simulink library "MarIn_blade"  (R2017a)
settings: Solver=VariableStepAuto  StartTime=0.0  StopTime=10.0  RelTol=1e-3
undefined symbols (not defined in the file or in its folder): bladePar, data_wind_mann, eta_init_n, g, k_t1, k_t2, k_w1, k_w2, lw2, m_h, meanWindSpeed, nu_init_b, p_h_dot_init, p_h_init, posCraneTip, posSling_b, posTuggerline_b, posTuggerlineBase_n, sigbuilder_block
undefined symbols (not defined in the file): d_w1, lt1_init
libraries: MarIn_blade x37
(part 2 of 2)

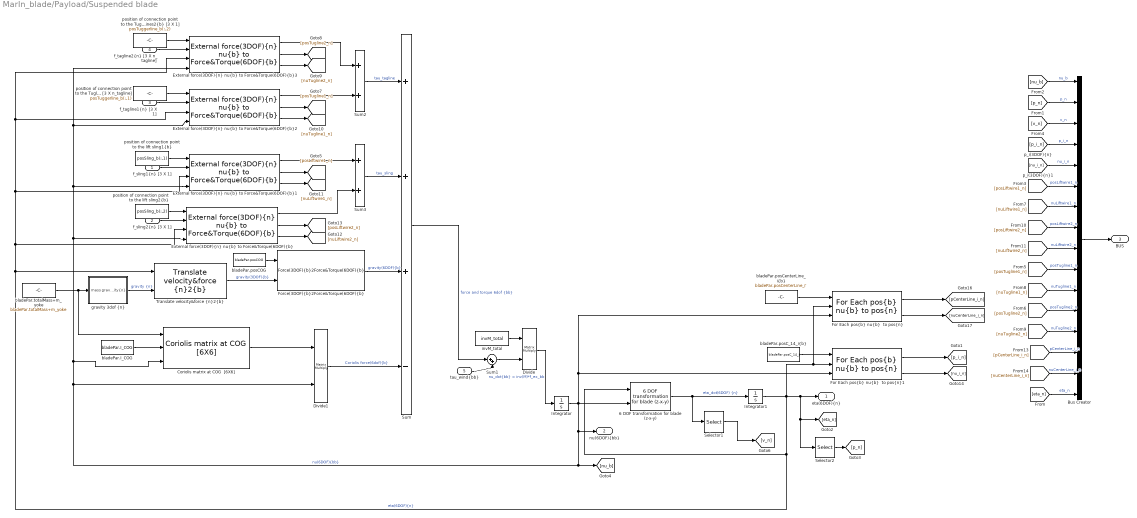
== system MarIn_blade/Payload/Suspended blade ==
  "f_sling1{n} [3 X 1]" : Inport
  "f_sling2{n} [3 X 1]" : Inport  Port=2
  "f_tagline1{n} [3 X 1]" : Inport  Port=3
  "f_tagline2{n} [3 X n_tagline]" : Inport  Port=4
  "tau_wind{bb}" : Inport  Port=5
  6 DOF transformation for blade (z-x-y) : MarIn_blade/Basic functions/6 DOF transformation for blade (z-x-y)
      settings: SourceProductName=MarIn(Blade)
  Bus Creator : BusCreator  Inputs=16
  Coriolis matrix at COG  [6X6] : MarIn_blade/Basic functions/Coriolis matrix at COG  [6X6]
      settings: SourceProductName=MarIn(Blade)
  Divide : Product  Inputs=**  Multiplication=Matrix(*)
  Divide1 : Product  Inputs=**  Multiplication=Matrix(*)
  External force(3DOF){n} nu{b} to Force&Torque(6DOF){b}{,1..3} (4 alike) : MarIn_blade/Basic functions/External force(3DOF){n} nu{b} to Force&Torque(6DOF){b}
      settings: SourceProductName=MarIn(Blade)
  "For Each pos{b} nu{b}  to pos{n}" : MarIn_blade/Basic functions/For Each pos{b} nu{b}  to pos{n}  posCOG_b=bladePar.posCOG  n_i=bladePar.n_i
      settings: SourceProductName=MarIn(Blade)
  "For Each pos{b} nu{b}  to pos{n}1" : MarIn_blade/Basic functions/For Each pos{b} nu{b}  to pos{n}  posCOG_b=bladePar.posCOG  n_i=bladePar.n_i
      settings: SourceProductName=MarIn(Blade)
  "Force(3DOF){b}2Force&Torque(6DOF){b}" : MarIn_blade/Basic functions/Force(3DOF){b}2Force&Torque(6DOF){b}  posCOG_bb=bladePar.posCOG
      settings: SourceProductName=MarIn(Blade)
  Integrator : Integrator  InitialCondition=nu_init_b
  Integrator1 : Integrator  InitialCondition=eta_init_n
  Selector1 : Selector  InputPortWidth=6  IndexOptions=Index vector (dialog)  Indices=[1 2 3]  OutputSizes=1
  Selector2 : Selector  InputPortWidth=6  IndexOptions=Index vector (dialog)  Indices=[1 2 3]  OutputSizes=1
  Sum : Sum  Inputs=+++-
  Sum1 : Sum  Inputs=|++
  Sum2 : Sum  Inputs=2
  Sum3 : Sum  Inputs=2
  "Translate velocity&force {n}2{b}" : MarIn_blade/Basic functions/Translate velocity&force {n}2{b}
      settings: SourceProductName=MarIn(Blade)
  bladePar.I_COG : Constant  Value=bladePar.I_COG
  bladePar.posCOG : Constant  Value=bladePar.posCOG
  "bladePar.posC_14_i{b}" : Constant  Value=bladePar.posC_14_i
  "bladePar.posCenterLine_i{b}" : Constant  Value=bladePar.posCenterLine_i'
  bladePar.totalMass+m_yoke : Constant  Value=bladePar.totalMass+m_yoke
  "gravity 3dof {n}" : Subsystem
  invM_total : Constant  Value=invM_total
  "position of connection point to the Tugline1{b} [3 X n_tagline]" : Constant  Value=posTuggerline_b(:,1)
  "position of connection point to the Tuglines2{b} [3 X 1]" : Constant  Value=posTuggerline_b(:,2)
  "position of connection point to the lift sling1{b}" : Constant  Value=posSling_b(:,1)
  "position of connection point to the lift sling2{b}" : Constant  Value=posSling_b(:,2)
  "eta(6DOF){n}" : Outport
  "nu(6DOF){bb}" : Outport  Port=2
  BUS : Outport  Port=3
  wires:
  [nuCenterLine_i_n] -> Bus Creator/15  "nuCenterLine_i_n"
  [pCenterLine_i_n] -> Bus Creator/14  "pCenterLine_i_n"
  Integrator/1 -> 6 DOF transformation for blade (z-x-y)/2, Divide1/2, Coriolis matrix at COG  [6X6]/3, "External force(3DOF){n} nu{b} to Force&Torque(6DOF){b}"/4, "External force(3DOF){n} nu{b} to Force&Torque(6DOF){b}1"/4, "External force(3DOF){n} nu{b} to Force&Torque(6DOF){b}3"/4, "External force(3DOF){n} nu{b} to Force&Torque(6DOF){b}2"/4, [nu_b], "nu(6DOF){bb}"/1, "For Each pos{b} nu{b}  to pos{n}1"/3, "For Each pos{b} nu{b}  to pos{n}"/3  "nu(6DOF){bb}"
  Integrator1/1 -> "eta(6DOF){n}"/1, [eta_n], Selector2/1, 6 DOF transformation for blade (z-x-y)/1, "Translate velocity&force {n}2{b}"/1, "External force(3DOF){n} nu{b} to Force&Torque(6DOF){b}"/3, "External force(3DOF){n} nu{b} to Force&Torque(6DOF){b}1"/3, "External force(3DOF){n} nu{b} to Force&Torque(6DOF){b}3"/3, "External force(3DOF){n} nu{b} to Force&Torque(6DOF){b}2"/3, "For Each pos{b} nu{b}  to pos{n}1"/2, "For Each pos{b} nu{b}  to pos{n}"/2  "eta(6DOF){n}"
  "For Each pos{b} nu{b}  to pos{n}"/1 -> [pCenterLine_i_n]
  "For Each pos{b} nu{b}  to pos{n}"/2 -> [nuCenterLine_i_n]
  "bladePar.posCenterLine_i{b}"/1 -> "For Each pos{b} nu{b}  to pos{n}"/1
  "bladePar.posC_14_i{b}"/1 -> "For Each pos{b} nu{b}  to pos{n}1"/1
  [nuLiftwire2_n] -> Bus Creator/9  "nuLiftwire2_n"
  [posLiftwire2_n] -> Bus Creator/8  "posLiftwire2_n"
  [nu_i_n] -> Bus Creator/5  "nu_i_n"
  "For Each pos{b} nu{b}  to pos{n}1"/2 -> [nu_i_n]
  "For Each pos{b} nu{b}  to pos{n}1"/1 -> [p_i_n]
  "External force(3DOF){n} nu{b} to Force&Torque(6DOF){b}"/3 -> [nuLiftwire2_n]
  "External force(3DOF){n} nu{b} to Force&Torque(6DOF){b}"/2 -> [posLiftwire2_n]
  "position of connection point to the lift sling2{b}"/1 -> "External force(3DOF){n} nu{b} to Force&Torque(6DOF){b}"/1
  "f_sling2{n} [3 X 1]"/1 -> "External force(3DOF){n} nu{b} to Force&Torque(6DOF){b}"/2
  Sum3/1 -> Sum/2  "tau_sling"
  [nuTugline2_n] -> Bus Creator/13  "nuTugline2_n"
  [nuTugline1_n] -> Bus Creator/11  "nuTugline1_n"
  [nuLiftwire1_n] -> Bus Creator/7  "nuLiftwire1_n"
  "External force(3DOF){n} nu{b} to Force&Torque(6DOF){b}1"/3 -> [nuLiftwire1_n]
  "External force(3DOF){n} nu{b} to Force&Torque(6DOF){b}2"/3 -> [nuTugline1_n]
  "External force(3DOF){n} nu{b} to Force&Torque(6DOF){b}3"/3 -> [nuTugline2_n]
  [posTugline2_n] -> Bus Creator/12  "posTugline2_n"
  "External force(3DOF){n} nu{b} to Force&Torque(6DOF){b}3"/2 -> [posTugline2_n]
  "External force(3DOF){n} nu{b} to Force&Torque(6DOF){b}3"/1 -> Sum2/1
  "f_tagline2{n} [3 X n_tagline]"/1 -> "External force(3DOF){n} nu{b} to Force&Torque(6DOF){b}3"/2
  "position of connection point to the Tuglines2{b} [3 X 1]"/1 -> "External force(3DOF){n} nu{b} to Force&Torque(6DOF){b}3"/1
  Sum2/1 -> Sum/1  "tau_tagline"
  "External force(3DOF){n} nu{b} to Force&Torque(6DOF){b}1"/1 -> Sum3/1
  "External force(3DOF){n} nu{b} to Force&Torque(6DOF){b}2"/2 -> [posTugline1_n]
  [posTugline1_n] -> Bus Creator/10  "posTugline1_n"
  Bus Creator/1 -> BUS/1
  [v_n] -> Bus Creator/3  "v_n"
  [posLiftwire1_n] -> Bus Creator/6  "posLiftwire1_n"
  [p_i_n] -> Bus Creator/4  "p_i_n"
  "External force(3DOF){n} nu{b} to Force&Torque(6DOF){b}1"/2 -> [posLiftwire1_n]
  [nu_b] -> Bus Creator/1  "nu_b"
  [p_n] -> Bus Creator/2  "p_n"
  Selector1/1 -> [v_n]
  Sum1/1 -> Divide/2
  "tau_wind{bb}"/1 -> Sum1/2
  "External force(3DOF){n} nu{b} to Force&Torque(6DOF){b}2"/1 -> Sum2/2
  "f_tagline1{n} [3 X 1]"/1 -> "External force(3DOF){n} nu{b} to Force&Torque(6DOF){b}2"/2
  "position of connection point to the Tugline1{b} [3 X n_tagline]"/1 -> "External force(3DOF){n} nu{b} to Force&Torque(6DOF){b}2"/1
  "position of connection point to the lift sling1{b}"/1 -> "External force(3DOF){n} nu{b} to Force&Torque(6DOF){b}1"/1
  invM_total/1 -> Divide/1
  bladePar.posCOG/1 -> "Force(3DOF){b}2Force&Torque(6DOF){b}"/1
  "Translate velocity&force {n}2{b}"/1 -> "Force(3DOF){b}2Force&Torque(6DOF){b}"/2  "gravity(3DOF){b}"
  "f_sling1{n} [3 X 1]"/1 -> "External force(3DOF){n} nu{b} to Force&Torque(6DOF){b}1"/2
  6 DOF transformation for blade (z-x-y)/1 -> Selector1/1, Integrator1/1  "eta_dot(6DOF) {n}"
  "gravity 3dof {n}"/1("gravity{n}") -> "Translate velocity&force {n}2{b}"/2  "gravity {n}"
  "Force(3DOF){b}2Force&Torque(6DOF){b}"/1 -> Sum/3  "gravity(6DOF){b}"
  bladePar.I_COG/1 -> Coriolis matrix at COG  [6X6]/2
  bladePar.totalMass+m_yoke/1 -> Coriolis matrix at COG  [6X6]/1, "gravity 3dof {n}"/1(mass)
  Divide/1 -> Integrator/1  "nu_dot{bb} = inv(M)*f_ex_bb"
  Divide1/1 -> Sum/4  "Coriolis force(6dof){b}"
  Coriolis matrix at COG  [6X6]/1 -> Divide1/1
  Sum/1 -> Sum1/1  "force and torque 6dof {bb}"
  "External force(3DOF){n} nu{b} to Force&Torque(6DOF){b}"/1 -> Sum3/2
  Selector2/1 -> [p_n]
  [eta_n] -> Bus Creator/16  "eta_n"

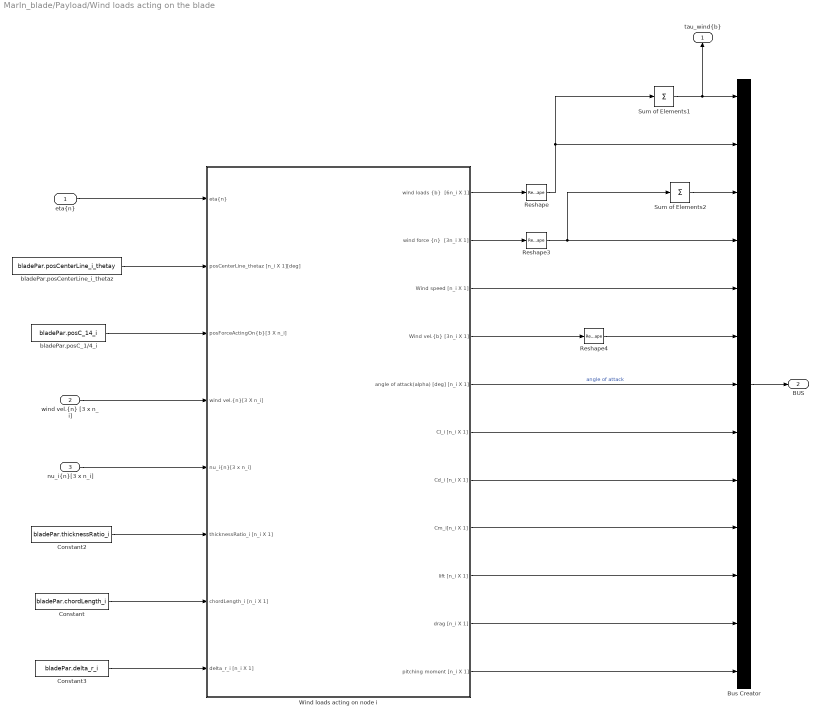
== system MarIn_blade/Payload/Wind loads acting on the blade ==
  "eta{n}" : Inport
  "wind vel.{n} [3 x n_i]" : Inport  Port=2
  "nu_i{n}[3 x n_i]" : Inport  Port=3
  Bus Creator : BusCreator  Inputs=13
  Constant : Constant  Value=bladePar.chordLength_i
  Constant2 : Constant  Value=bladePar.thicknessRatio_i
  Constant3 : Constant  Value=bladePar.delta_r_i
  Reshape : Reshape  OutputDimensionality=Customize  OutputDimensions=[6,length(bladePar.chordLength_i)]
  Reshape3 : Reshape  OutputDimensionality=Customize  OutputDimensions=[3,length(bladePar.chordLength_i)]
  Reshape4 : Reshape  OutputDimensionality=Customize  OutputDimensions=[3,length(bladePar.chordLength_i)]
  Sum of Elements1 : Sum  Inputs=+  CollapseMode=Specified dimension  CollapseDim=2
  Sum of Elements2 : Sum  Inputs=+  CollapseMode=Specified dimension  CollapseDim=2
  Wind loads acting on node i : Subsystem
  bladePar.posC_1/4_i : Constant  Value=bladePar.posC_14_i
  bladePar.posCenterLine_i_thetaz : Constant  Value=bladePar.posCenterLine_i_thetay
  "tau_wind{b}" : Outport
  BUS : Outport  Port=2
  wires:
  "eta{n}"/1 -> Wind loads acting on node i/1("eta{n}")
  Wind loads acting on node i/6(Cl_i [n_i X 1]) -> Bus Creator/8
  "wind vel.{n} [3 x n_i]"/1 -> Wind loads acting on node i/4("wind vel.{n}[3 X n_i]")
  Constant/1 -> Wind loads acting on node i/7(chordLength_i [n_i X 1])
  Wind loads acting on node i/3(Wind speed [n_i X 1]) -> Bus Creator/5
  Wind loads acting on node i/5("angle of attack(alpha) [deg] [n_i X 1] ") -> Bus Creator/7  "angle of attack"
  bladePar.posCenterLine_i_thetaz/1 -> Wind loads acting on node i/2(posCenterLine_thetaz [n_i X 1][deg])
  bladePar.posC_1/4_i/1 -> Wind loads acting on node i/3("posForceActingOn{b}[3 X n_i]")
  Wind loads acting on node i/1("wind loads {b}  [6n_i X 1]") -> Reshape/1
  Constant2/1 -> Wind loads acting on node i/6(thicknessRatio_i [n_i X 1])
  Constant3/1 -> Wind loads acting on node i/8(delta_r_i [n_i X 1])
  Reshape/1 -> Sum of Elements1/1, Bus Creator/2
  Wind loads acting on node i/4("Wind vel.{b} [3n_i X 1] ") -> Reshape4/1
  Bus Creator/1 -> BUS/1
  Wind loads acting on node i/11(pitching moment [n_i X 1]) -> Bus Creator/13
  Reshape3/1 -> Sum of Elements2/1, Bus Creator/4
  Wind loads acting on node i/10(drag [n_i X 1]) -> Bus Creator/12
  Wind loads acting on node i/8(Cm_i[n_i X 1]) -> Bus Creator/10
  Wind loads acting on node i/9(lift [n_i X 1]) -> Bus Creator/11
  Sum of Elements2/1 -> Bus Creator/3
  Wind loads acting on node i/2("wind force {n}  [3n_i X 1]") -> Reshape3/1
  Wind loads acting on node i/7(Cd_i [n_i X 1]) -> Bus Creator/9
  Reshape4/1 -> Bus Creator/6
  Sum of Elements1/1 -> Bus Creator/1, "tau_wind{b}"/1
  "nu_i{n}[3 x n_i]"/1 -> Wind loads acting on node i/5("nu_i{n}[3 x n_i]")

== system MarIn_blade/[Example] Single blade installation/More Info1 ==

== system MarIn_blade/[Example] Single blade installation/Signal Builder1 ==
  Demux : Demux  Tag=STV Demux  Outputs=1
  FromWs : FromWorkspace  Tag=STV FromWs  VariableName=tuvar  SampleTime=0
      SigBuilderData=|
      | common.afterFinalStr = 'Extrapolate'
      | common.sampleTime = 0
      | dataSet.timeRange = [0 3000]
      | dataSet.name = 'Group 1'
      | sbobj.Groups.Name = 'Group 1'
      | sbobj.Groups.Signals.Name = 'Signal 2'
      | sbobj.Groups.Signals.XData = [0 10 30 90 3000]
      | sbobj.Groups.Signals.YData = [0 0 -0.04 0 0]
      | sbobj.Groups.TimeRange = [0 3000]
  Signal 2 : Outport  Tag=STV Outport
  wires:
  FromWs/1 -> Demux/1
  Demux/1 -> Signal 2/1

== system MarIn_blade/[Example] Single blade installation/wind ramp ==
  Demux : Demux  Tag=STV Demux  Outputs=1
  FromWs : FromWorkspace  Tag=STV FromWs  VariableName=tuvar  SampleTime=0
      SigBuilderData=|
      | common.afterFinalStr = 'Extrapolate'
      | common.sampleTime = 0
      | dataSet.timeRange = [0 3000]
      | dataSet.name = 'Group 1'
      | sbobj.Groups.Name = 'Group 1'
      | sbobj.Groups.Signals.Name = 'Signal 1'
      | sbobj.Groups.Signals.XData = [0 1 5 3000]
      | sbobj.Groups.Signals.YData = [0 0 1 1]
      | sbobj.Groups.TimeRange = [0 3000]
  Signal 1 : Outport  Tag=STV Outport
  wires:
  FromWs/1 -> Demux/1
  Demux/1 -> Signal 1/1

== system MarIn_blade/Basic functions/3x3 Cross Product C=AxB/Subsystem2 ==
  A : Inport
  B : Inport  Port=2
  Demux : Demux  Outputs=3
  Demux1 : Demux  Outputs=3
  Mux : Mux  Inputs=3
  i x j : Product  SaturateOnIntegerOverflow=on  InputSameDT=on  OutDataTypeStr=Inherit: Same as first input
  j x k : Product  SaturateOnIntegerOverflow=on  InputSameDT=on  OutDataTypeStr=Inherit: Same as first input
  k x i : Product  SaturateOnIntegerOverflow=on  InputSameDT=on  OutDataTypeStr=Inherit: Same as first input
  Out1 : Outport
  wires:
  Demux1/3 -> j x k/2
  Demux/2 -> j x k/1
  Demux/3 -> k x i/1
  Demux1/1 -> k x i/2
  Demux1/2 -> i x j/2
  Demux/1 -> i x j/1
  i x j/1 -> Mux/3
  k x i/1 -> Mux/2
  j x k/1 -> Mux/1
  B/1 -> Demux1/1
  A/1 -> Demux/1
  Mux/1 -> Out1/1

== system MarIn_blade/Basic functions/3x3 Cross Product C=AxB/Subsystem3 ==
  A : Inport
  B : Inport  Port=2
  Demux2 : Demux  Outputs=3
  Demux3 : Demux  Outputs=3
  Mux1 : Mux  Inputs=3
  i x k : Product  SaturateOnIntegerOverflow=on  InputSameDT=on  OutDataTypeStr=Inherit: Same as first input
  j x i : Product  SaturateOnIntegerOverflow=on  InputSameDT=on  OutDataTypeStr=Inherit: Same as first input
  k x j : Product  SaturateOnIntegerOverflow=on  InputSameDT=on  OutDataTypeStr=Inherit: Same as first input
  Out1 : Outport
  wires:
  B/1 -> Demux3/1
  A/1 -> Demux2/1
  Mux1/1 -> Out1/1
  j x i/1 -> Mux1/3
  i x k/1 -> Mux1/2
  k x j/1 -> Mux1/1
  Demux3/1 -> j x i/2
  Demux2/2 -> j x i/1
  Demux3/3 -> i x k/2
  Demux2/1 -> i x k/1
  Demux3/2 -> k x j/2
  Demux2/3 -> k x j/1

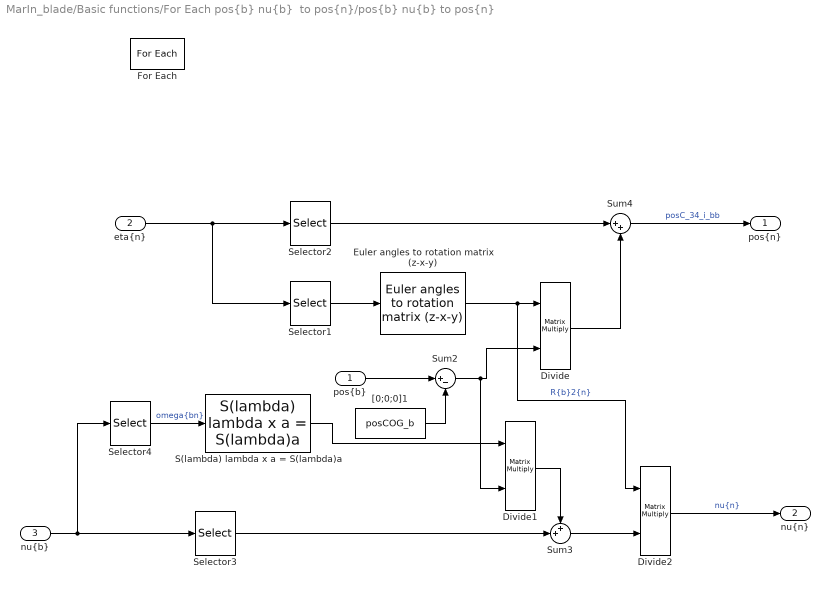
== system MarIn_blade/Basic functions/For Each pos{b} nu{b}  to pos{n}/pos{b} nu{b} to pos{n} ==
  "pos{b}" : Inport  Partition=on  PartitionDimension=2  PartitionWidth=1
  "eta{n}" : Inport  Port=2
  "nu{b}" : Inport  Port=3
  Divide : Product  Inputs=**  Multiplication=Matrix(*)
  Divide1 : Product  Multiplication=Matrix(*)
  Divide2 : Product  Multiplication=Matrix(*)
  Euler angles to rotation matrix (z-x-y) : MarIn_blade/Basic functions/Euler angles to rotation matrix (z-x-y)
      settings: SourceProductName=MarIn(Blade)
  For Each : ForEach  DisableCoverage=on  IndexMode=One-based
  S(lambda) lambda x a = S(lambda)a : MarIn_blade/Basic functions/S(lambda) lambda x a = S(lambda)a
      settings: SourceProductName=MarIn (Blade)
  Selector1 : Selector  InputPortWidth=6  IndexOptions=Index vector (dialog)  Indices=[4 5 6]  OutputSizes=1
  Selector2 : Selector  InputPortWidth=6  IndexOptions=Index vector (dialog)  Indices=[1 2 3]  OutputSizes=1
  Selector3 : Selector  InputPortWidth=6  IndexOptions=Index vector (dialog)  Indices=[1 2 3]  OutputSizes=1
  Selector4 : Selector  InputPortWidth=6  IndexOptions=Index vector (dialog)  Indices=[4 5 6]  OutputSizes=1
  Sum2 : Sum  Inputs=|+-
  Sum3 : Sum  Inputs=++|
  Sum4 : Sum  Inputs=|++
  "[0;0;0]1" : Constant  Value=posCOG_b
  "pos{n}" : Outport  ConcatenationDimension=1
  "nu{n}" : Outport  Port=2  ConcatenationDimension=1
  wires:
  S(lambda) lambda x a = S(lambda)a/1 -> Divide1/1
  Divide1/1 -> Sum3/1
  Sum3/1 -> Divide2/2
  "[0;0;0]1"/1 -> Sum2/2
  Sum2/1 -> Divide/2, Divide1/2
  Divide2/1 -> "nu{n}"/1  "nu{n}"
  Selector3/1 -> Sum3/2
  "nu{b}"/1 -> Selector4/1, Selector3/1
  "pos{b}"/1 -> Sum2/1
  Divide/1 -> Sum4/2
  Euler angles to rotation matrix (z-x-y)/1 -> Divide2/1, Divide/1  "R{b}2{n}"
  Selector2/1 -> Sum4/1
  "eta{n}"/1 -> Selector2/1, Selector1/1
  Sum4/1 -> "pos{n}"/1  "posC_34_i_bb"
  Selector1/1 -> Euler angles to rotation matrix (z-x-y)/1
  Selector4/1 -> S(lambda) lambda x a = S(lambda)a/1  "omega{bn}"

== system MarIn_blade/Basic functions/Force(3DOF){b}2Force&Torque(6DOF){b}/3x3 Cross Product C=AxB ==
  A : Inport
  B : Inport  Port=2
  "A " : InportShadow
  "B " : InportShadow  Port=2
  Subsystem2 : Subsystem
  Subsystem3 : Subsystem
  Sum : Sum  Inputs=+|-  SaturateOnIntegerOverflow=on  InputSameDT=on  OutDataTypeStr=Inherit: Same as first input
  C : Outport
  wires:
  Subsystem3/1(Out1) -> Sum/2
  Subsystem2/1(Out1) -> Sum/1
  A/1 -> Subsystem2/1(A)
  B/1 -> Subsystem2/2(B)
  Sum/1 -> C/1
  "A "/1 -> Subsystem3/1(A)
  "B "/1 -> Subsystem3/2(B)

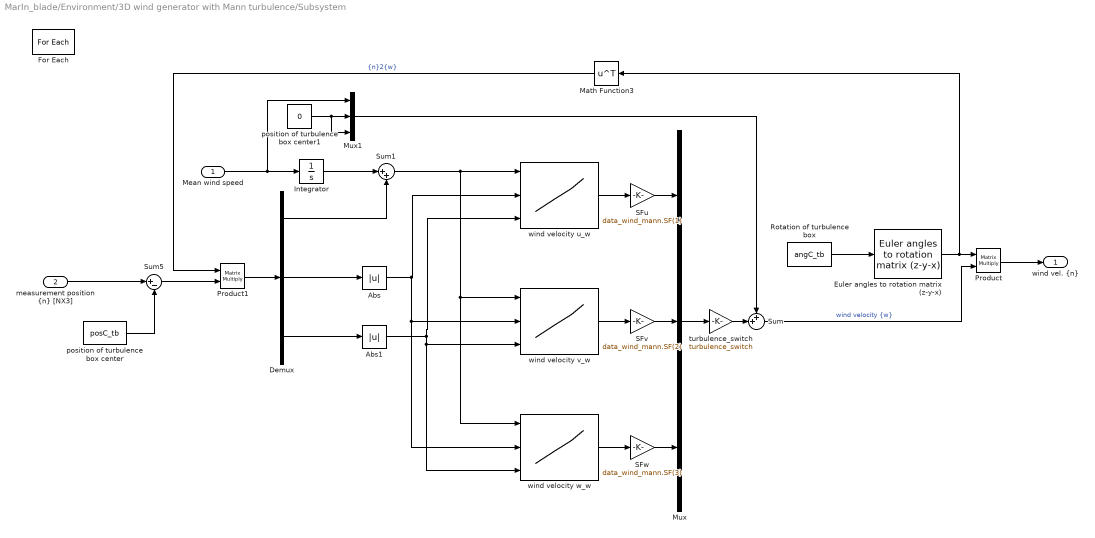
== system MarIn_blade/Environment/3D wind generator with Mann turbulence/Subsystem ==
  Mean wind speed : Inport
  "measurement position {n} [NX3]" : Inport  Port=2  Partition=on  PartitionDimension=2  PartitionWidth=1
  Abs : Abs
  Abs1 : Abs
  Demux : Demux  Outputs=3
  Euler angles to rotation matrix (z-y-x) : MarIn_blade/Basic functions/Euler angles to rotation matrix (z-y-x)
      settings: SourceProductName=MarIn(Blade)
  For Each : ForEach  DisableCoverage=on  IndexMode=One-based
  Integrator : Integrator
  Math Function3 : Math  Operator=transpose  SaturateOnIntegerOverflow=on
  Mux : Mux  Inputs=3
  Mux1 : Mux  Inputs=3
  Product : Product  Multiplication=Matrix(*)
  Product1 : Product  Multiplication=Matrix(*)
  Rotation of turbulence box : Constant  Value=angC_tb
  SFu : Gain  Gain=data_wind_mann.SF(1)
  SFv : Gain  Gain=data_wind_mann.SF(2)
  SFw : Gain  Gain=data_wind_mann.SF(3)
  Sum : Sum  Inputs=++|
  Sum1 : Sum  Inputs=|++
  Sum5 : Sum  Inputs=|+-
  position of turbulence box center : Constant  Value=posC_tb
  position of turbulence box center1 : Constant  Value=0
  turbulence_switch : Gain  Gain=turbulence_switch
  wind velocity u_w : Lookup_n-D  NumberOfTableDimensions=3  BreakpointsForDimension1=data_wind_mann.posX  BreakpointsForDimension2=data_wind_mann.posY  BreakpointsForDimension3=data_wind_mann.posZ  Table=data_wind_mann.u  InternalRulePriority=Speed  RndMeth=Simplest  InputSameDT=on
  wind velocity v_w : Lookup_n-D  NumberOfTableDimensions=3  BreakpointsForDimension1=data_wind_mann.posX  BreakpointsForDimension2=data_wind_mann.posY  BreakpointsForDimension3=data_wind_mann.posZ  Table=data_wind_mann.v  InternalRulePriority=Speed  RndMeth=Simplest  InputSameDT=on
  wind velocity w_w : Lookup_n-D  NumberOfTableDimensions=3  BreakpointsForDimension1=data_wind_mann.posX  BreakpointsForDimension2=data_wind_mann.posY  BreakpointsForDimension3=data_wind_mann.posZ  Table=data_wind_mann.w  InternalRulePriority=Speed  RndMeth=Simplest  InputSameDT=on
  "wind vel. {n}" : Outport  ConcatenationDimension=1
  wires:
  Product/1 -> "wind vel. {n}"/1
  Demux/2 -> Abs/1
  "measurement position {n} [NX3]"/1 -> Sum5/1
  Sum/1 -> Product/2  "wind velocity {w}"
  SFu/1 -> Mux/1
  Sum1/1 -> wind velocity w_w/1, wind velocity v_w/1, wind velocity u_w/1
  Rotation of turbulence box/1 -> Euler angles to rotation matrix (z-y-x)/1
  Sum5/1 -> Product1/2
  Euler angles to rotation matrix (z-y-x)/1 -> Math Function3/1, Product/1
  Demux/1 -> Sum1/2
  wind velocity u_w/1 -> SFu/1
  position of turbulence box center1/1 -> Mux1/3, Mux1/2
  Math Function3/1 -> Product1/1  "{n}2{w}"
  Mux1/1 -> Sum/1
  Mux/1 -> turbulence_switch/1
  SFv/1 -> Mux/2
  wind velocity v_w/1 -> SFv/1
  Product1/1 -> Demux/1
  turbulence_switch/1 -> Sum/2
  Abs1/1 -> wind velocity w_w/3, wind velocity v_w/3, wind velocity u_w/3
  position of turbulence box center/1 -> Sum5/2
  SFw/1 -> Mux/3
  Abs/1 -> wind velocity w_w/2, wind velocity v_w/2, wind velocity u_w/2
  Integrator/1 -> Sum1/1
  Mean wind speed/1 -> Integrator/1, Mux1/1
  wind velocity w_w/1 -> SFw/1
  Demux/3 -> Abs1/1

== system MarIn_blade/Payload/Suspended blade/gravity 3dof {n} ==
  mass : Inport
  Constant : Constant  Value=0
  Gain : Gain  Gain=9.81
  Mux : Mux  Inputs=3
  "gravity{n}" : Outport
  wires:
  Gain/1 -> Mux/3
  Constant/1 -> Mux/2, Mux/1
  Mux/1 -> "gravity{n}"/1  "Gravity"
  mass/1 -> Gain/1

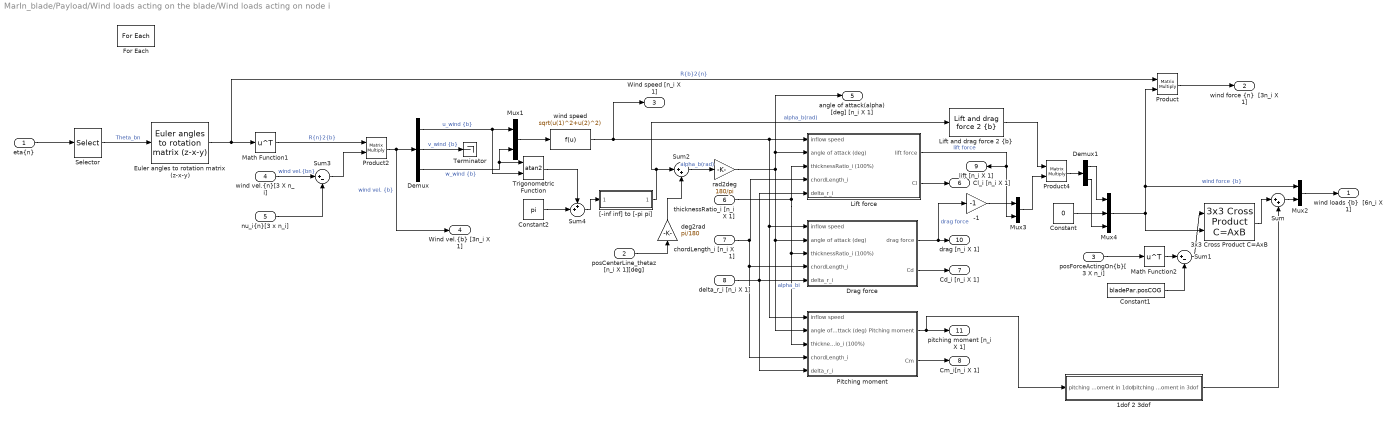
== system MarIn_blade/Payload/Wind loads acting on the blade/Wind loads acting on node i ==
  "eta{n}" : Inport
  posCenterLine_thetaz [n_i X 1][deg] : Inport  Port=2  Partition=on  PartitionDimension=1  PartitionWidth=1
  "posForceActingOn{b}[3 X n_i]" : Inport  Port=3  Partition=on  PartitionDimension=2  PartitionWidth=1
  "wind vel.{n}[3 X n_i]" : Inport  Port=4  Partition=on  PartitionDimension=2  PartitionWidth=1
  "nu_i{n}[3 x n_i]" : Inport  Port=5  Partition=on  PartitionDimension=2  PartitionWidth=1
  thicknessRatio_i [n_i X 1] : Inport  Port=6  Partition=on  PartitionDimension=1  PartitionWidth=1
  chordLength_i [n_i X 1] : Inport  Port=7  Partition=on  PartitionDimension=1  PartitionWidth=1
  delta_r_i [n_i X 1] : Inport  Port=8  Partition=on  PartitionDimension=1  PartitionWidth=1
  -1 : Gain  Gain=-1
  1dof 2 3dof : Subsystem
  3x3 Cross Product C=AxB : MarIn_blade/Basic functions/3x3 Cross Product C=AxB
      settings: SourceProductName=MarIn(Blade)
  Constant : Constant  Value=0
  Constant1 : Constant  Value=bladePar.posCOG
  Constant2 : Constant  Value=pi
  Demux : Demux  Outputs=3
  Demux1 : Demux  Outputs=2
  Drag force : Subsystem
  Euler angles to rotation matrix (z-x-y) : MarIn_blade/Basic functions/Euler angles to rotation matrix (z-x-y)
      settings: SourceProductName=MarIn(Blade)
  For Each : ForEach  DisableCoverage=on  IndexMode=One-based
  "Lift and drag force 2 {b}" : MarIn_blade/Basic functions/Lift and drag force 2 {b}
      settings: SourceProductName=MarIn(Blade)
  Lift force : Subsystem
  Math Function1 : Math  Operator=transpose  SaturateOnIntegerOverflow=on
  Math Function2 : Math  Operator=transpose  SaturateOnIntegerOverflow=on
  Mux1 : Mux  Inputs=2
  Mux2 : Mux  Inputs=2
  Mux3 : Mux  Inputs=2
  Mux4 : Mux  Inputs=3
  Pitching moment : Subsystem
  Product : Product  Multiplication=Matrix(*)
  Product2 : Product  Multiplication=Matrix(*)
  Product4 : Product  Multiplication=Matrix(*)
  Selector : Selector  InputPortWidth=6  IndexOptions=Index vector (dialog)  Indices=[4 5 6]  OutputSizes=1
  Sum : Sum  Inputs=|++
  Sum1 : Sum  Inputs=|+-
  Sum2 : Sum  Inputs=|++
  Sum3 : Sum  Inputs=|+-
  Sum4 : Sum  Inputs=++|
  Terminator : Terminator
  Trigonometric Function : Trigonometry  Operator=atan2
  "[-inf inf] to [-pi pi]" : Subsystem  mask([-inf inf] to [-pi pi]){}
      mask help: Converts an angle in rad to (-pi pi)
  deg2rad : Gain  Gain=pi/180
  rad2deg : Gain  Gain=180/pi
  wind speed : Fcn  Expr=sqrt(u(1)^2+u(2)^2)
  "wind loads {b}  [6n_i X 1]" : Outport  ConcatenationDimension=1
  "wind force {n}  [3n_i X 1]" : Outport  Port=2  ConcatenationDimension=1
  Wind speed [n_i X 1] : Outport  Port=3  ConcatenationDimension=1
  "Wind vel.{b} [3n_i X 1] " : Outport  Port=4  ConcatenationDimension=1
  "angle of attack(alpha) [deg] [n_i X 1] " : Outport  Port=5  ConcatenationDimension=1
  Cl_i [n_i X 1] : Outport  Port=6  ConcatenationDimension=1
  Cd_i [n_i X 1] : Outport  Port=7  ConcatenationDimension=1
  Cm_i[n_i X 1] : Outport  Port=8  ConcatenationDimension=1
  lift [n_i X 1] : Outport  Port=9  ConcatenationDimension=1
  drag [n_i X 1] : Outport  Port=10  ConcatenationDimension=1
  pitching moment [n_i X 1] : Outport  Port=11  ConcatenationDimension=1
  wires:
  posCenterLine_thetaz [n_i X 1][deg]/1 -> deg2rad/1
  "eta{n}"/1 -> Selector/1
  Selector/1 -> Euler angles to rotation matrix (z-x-y)/1  "Theta_bn"
  Math Function1/1 -> Product2/1  "R{n}2{b}"
  Product2/1 -> "Wind vel.{b} [3n_i X 1] "/1, Demux/1  "wind vel. {b}"
  Lift force/1(lift force) -> Mux3/2, lift [n_i X 1]/1  "lift force"
  Demux/1 -> Trigonometric Function/2, Mux1/1  "u_wind {b}"
  Demux/3 -> Mux1/2, Trigonometric Function/1  "w_wind {b}"
  Demux/2 -> Terminator/1  "v_wind {b}"
  Mux1/1 -> wind speed/1
  wind speed/1 -> Pitching moment/1(inflow speed), Drag force/1(inflow speed), Lift force/1(inflow speed), Wind speed [n_i X 1]/1
  rad2deg/1 -> Lift force/2(angle of attack (deg)), "angle of attack(alpha) [deg] [n_i X 1] "/1, Pitching moment/2(angle of attack (deg)), Drag force/2(angle of attack (deg))  "alpha_bi"
  Sum1/1 -> 3x3 Cross Product C=AxB/1
  Mux4/1 -> 3x3 Cross Product C=AxB/2, Mux2/1, Product/2  "wind force {b}"
  "posForceActingOn{b}[3 X n_i]"/1 -> Math Function2/1
  Constant1/1 -> Sum1/2
  thicknessRatio_i [n_i X 1]/1 -> Pitching moment/3(thicknessRatio_i (100%)), Drag force/3(thicknessRatio_i (100%)), Lift force/3(thicknessRatio_i (100%))
  chordLength_i [n_i X 1]/1 -> Pitching moment/4(chordLength_i), Drag force/4(chordLength_i), Lift force/4(chordLength_i)
  delta_r_i [n_i X 1]/1 -> Drag force/5(delta_r_i), Pitching moment/5(delta_r_i), Lift force/5(delta_r_i)
  Math Function2/1 -> Sum1/1
  Euler angles to rotation matrix (z-x-y)/1 -> Product/1, Math Function1/1  "R{b}2{n}"
  "wind vel.{n}[3 X n_i]"/1 -> Sum3/1  "wind vel.{bn}"
  Sum3/1 -> Product2/2
  Lift force/2(Cl) -> Cl_i [n_i X 1]/1
  Drag force/2(Cd) -> Cd_i [n_i X 1]/1
  Sum2/1 -> rad2deg/1  "alpha_b(rad)"
  Pitching moment/1(Pitching moment) -> 1dof 2 3dof/1("pitching moment in 1dof "), pitching moment [n_i X 1]/1
  Pitching moment/2(Cm) -> Cm_i[n_i X 1]/1
  Drag force/1(drag force) -> -1/1, drag [n_i X 1]/1  "drag force"
  Product/1 -> "wind force {n}  [3n_i X 1]"/1
  1dof 2 3dof/1(pitching moment in 3dof) -> Sum/2
  Mux2/1 -> "wind loads {b}  [6n_i X 1]"/1
  3x3 Cross Product C=AxB/1 -> Sum/1
  Sum/1 -> Mux2/2
  Trigonometric Function/1 -> Sum4/1
  -1/1 -> Mux3/1
  Product4/1 -> Demux1/1
  Constant/1 -> Mux4/2
  "Lift and drag force 2 {b}"/1 -> Product4/1
  Mux3/1 -> Product4/2
  "nu_i{n}[3 x n_i]"/1 -> Sum3/2
  Sum4/1 -> "[-inf inf] to [-pi pi]"/1(x [-inf inf])
  Demux1/1 -> Mux4/1
  Demux1/2 -> Mux4/3
  deg2rad/1 -> Sum2/2
  Constant2/1 -> Sum4/2
  "[-inf inf] to [-pi pi]"/1(y [-pi pi]) -> "Lift and drag force 2 {b}"/1, Sum2/1  "alpha_b(rad)"

== system MarIn_blade/Basic functions/Force(3DOF){b}2Force&Torque(6DOF){b}/3x3 Cross Product C=AxB/Subsystem2 ==
  A : Inport
  B : Inport  Port=2
  Demux : Demux  Outputs=3
  Demux1 : Demux  Outputs=3
  Mux : Mux  Inputs=3
  i x j : Product  SaturateOnIntegerOverflow=on  InputSameDT=on  OutDataTypeStr=Inherit: Same as first input
  j x k : Product  SaturateOnIntegerOverflow=on  InputSameDT=on  OutDataTypeStr=Inherit: Same as first input
  k x i : Product  SaturateOnIntegerOverflow=on  InputSameDT=on  OutDataTypeStr=Inherit: Same as first input
  Out1 : Outport
  wires:
  Mux/1 -> Out1/1
  A/1 -> Demux/1
  B/1 -> Demux1/1
  j x k/1 -> Mux/1
  k x i/1 -> Mux/2
  i x j/1 -> Mux/3
  Demux/1 -> i x j/1
  Demux1/2 -> i x j/2
  Demux1/1 -> k x i/2
  Demux/3 -> k x i/1
  Demux/2 -> j x k/1
  Demux1/3 -> j x k/2

== system MarIn_blade/Basic functions/Force(3DOF){b}2Force&Torque(6DOF){b}/3x3 Cross Product C=AxB/Subsystem3 ==
  A : Inport
  B : Inport  Port=2
  Demux2 : Demux  Outputs=3
  Demux3 : Demux  Outputs=3
  Mux1 : Mux  Inputs=3
  i x k : Product  SaturateOnIntegerOverflow=on  InputSameDT=on  OutDataTypeStr=Inherit: Same as first input
  j x i : Product  SaturateOnIntegerOverflow=on  InputSameDT=on  OutDataTypeStr=Inherit: Same as first input
  k x j : Product  SaturateOnIntegerOverflow=on  InputSameDT=on  OutDataTypeStr=Inherit: Same as first input
  Out1 : Outport
  wires:
  Demux2/3 -> k x j/1
  Demux3/2 -> k x j/2
  Demux2/1 -> i x k/1
  Demux3/3 -> i x k/2
  Demux2/2 -> j x i/1
  Demux3/1 -> j x i/2
  k x j/1 -> Mux1/1
  i x k/1 -> Mux1/2
  j x i/1 -> Mux1/3
  Mux1/1 -> Out1/1
  A/1 -> Demux2/1
  B/1 -> Demux3/1

== system MarIn_blade/Payload/Wind loads acting on the blade/Wind loads acting on node i/1dof 2 3dof ==
  "pitching moment in 1dof " : Inport
  Constant3 : Constant  Value=0
  Mux : Mux  Inputs=3
  pitching moment in 3dof : Outport
  wires:
  Constant3/1 -> Mux/3, Mux/1
  Mux/1 -> pitching moment in 3dof/1
  "pitching moment in 1dof "/1 -> Mux/2

== system MarIn_blade/Payload/Wind loads acting on the blade/Wind loads acting on node i/Drag force ==
  inflow speed : Inport
  angle of attack (deg) : Inport  Port=2
  thicknessRatio_i (100%) : Inport  Port=3
  chordLength_i : Inport  Port=4
  delta_r_i : Inport  Port=5
  2-D Lookup Cd : Lookup_n-D  BreakpointsForDimension1=bladePar.data_Blade_clcdcm.alpha  BreakpointsForDimension2=bladePar.data_Blade_clcdcm.thickness  Table=bladePar.data_Blade_clcdcm.Cd  InternalRulePriority=Speed  RndMeth=Simplest  InputSameDT=on
  Gain1 : Gain  Gain=0.5
  Math Function : Math  Operator=square  SaturateOnIntegerOverflow=on
  Product2 : Product  Inputs=4
  Product3 : Product
  rho_air : Constant  Value=bladePar.rho_air
  drag force : Outport
  Cd : Outport  Port=2
  wires:
  2-D Lookup Cd/1 -> Cd/1, Product2/2
  Gain1/1 -> Product2/1
  Math Function/1 -> Product2/3
  rho_air/1 -> Gain1/1
  delta_r_i/1 -> Product3/2
  angle of attack (deg)/1 -> 2-D Lookup Cd/1
  chordLength_i/1 -> Product3/1
  inflow speed/1 -> Math Function/1
  Product3/1 -> Product2/4  "S wing area"
  Product2/1 -> drag force/1
  thicknessRatio_i (100%)/1 -> 2-D Lookup Cd/2

== system MarIn_blade/Payload/Wind loads acting on the blade/Wind loads acting on node i/Lift force ==
  inflow speed : Inport
  angle of attack (deg) : Inport  Port=2
  thicknessRatio_i (100%) : Inport  Port=3
  chordLength_i : Inport  Port=4
  delta_r_i : Inport  Port=5
  2-D Lookup Cl : Lookup_n-D  BreakpointsForDimension1=bladePar.data_Blade_clcdcm.alpha  BreakpointsForDimension2=bladePar.data_Blade_clcdcm.thickness  Table=bladePar.data_Blade_clcdcm.Cl  InternalRulePriority=Speed  RndMeth=Simplest  InputSameDT=on
  Gain : Gain  Gain=0.5
  Math Function : Math  Operator=square  SaturateOnIntegerOverflow=on
  Product : Product  Inputs=4
  Product1 : Product
  rho_air : Constant  Value=bladePar.rho_air
  lift force : Outport
  Cl : Outport  Port=2
  wires:
  Product1/1 -> Product/4  "S wing area"
  chordLength_i/1 -> Product1/1
  delta_r_i/1 -> Product1/2
  inflow speed/1 -> Math Function/1
  angle of attack (deg)/1 -> 2-D Lookup Cl/1
  rho_air/1 -> Gain/1
  Math Function/1 -> Product/3
  Gain/1 -> Product/1
  2-D Lookup Cl/1 -> Cl/1, Product/2
  Product/1 -> lift force/1
  thicknessRatio_i (100%)/1 -> 2-D Lookup Cl/2

== system MarIn_blade/Payload/Wind loads acting on the blade/Wind loads acting on node i/Pitching moment ==
  inflow speed : Inport
  angle of attack (deg) : Inport  Port=2
  thicknessRatio_i (100%) : Inport  Port=3
  chordLength_i : Inport  Port=4
  delta_r_i : Inport  Port=5
  2-D Lookup Cm : Lookup_n-D  BreakpointsForDimension1=bladePar.data_Blade_clcdcm.alpha  BreakpointsForDimension2=bladePar.data_Blade_clcdcm.thickness  Table=bladePar.data_Blade_clcdcm.Cm  InternalRulePriority=Speed  RndMeth=Simplest  InputSameDT=on
  Gain1 : Gain  Gain=0.5
  Math Function : Math  Operator=square  SaturateOnIntegerOverflow=on
  Product2 : Product  Inputs=4
  Product3 : Product  Inputs=3
  rho_air : Constant  Value=bladePar.rho_air
  Pitching moment : Outport
  Cm : Outport  Port=2
  wires:
  thicknessRatio_i (100%)/1 -> 2-D Lookup Cm/2
  Product2/1 -> Pitching moment/1
  Product3/1 -> Product2/4  "S wing area"
  inflow speed/1 -> Math Function/1
  chordLength_i/1 -> Product3/1, Product3/2
  angle of attack (deg)/1 -> 2-D Lookup Cm/1
  delta_r_i/1 -> Product3/3
  rho_air/1 -> Gain1/1
  Math Function/1 -> Product2/3
  Gain1/1 -> Product2/1
  2-D Lookup Cm/1 -> Product2/2, Cm/1

== system MarIn_blade/Payload/Wind loads acting on the blade/Wind loads acting on node i/[-inf inf] to [-pi pi] ==
  note: r
  note: x
  x [-inf inf] : Inport
  Constant : Constant  Value=2*pi
  Gain : Gain  Gain=pi  SaturateOnIntegerOverflow=on  OutDataTypeStr=Inherit: Same as input  ParamDataTypeStr=Inherit: Same as input
  Math Function : Math  Operator=rem  SaturateOnIntegerOverflow=on
  Saturation : Saturate  UpperLimit=1e10  LowerLimit=-1e10
  Sign : Signum
  Sum : Sum  Inputs=|+-  SaturateOnIntegerOverflow=on
  Sum1 : Sum  Inputs=|++  SaturateOnIntegerOverflow=on
  y [-pi pi] : Outport
  wires:
  Saturation/1 -> Sign/1, Sum1/1
  Sum/1 -> y [-pi pi]/1
  Math Function/1 -> Sum/1
  Constant/1 -> Math Function/2
  Sum1/1 -> Math Function/1
  Gain/1 -> Sum1/2, Sum/2
  Sign/1 -> Gain/1
  x [-inf inf]/1 -> Saturation/1
